simulink model "A1_acc"  (R2024a)
settings: Solver=ode45  StartTime=0.0  StopTime=80.0  MaxStep=0.001  RelTol=1e-3
values from neighbouring files (symbols this model uses):
  a = data(2)    [A1_10.m]    (also in problem6.m = 270)
  b = data(3)    [A1_10.m]    (also in problem6.m = 11000)
  kd = (0.155+3*p)/6.322    (= -0.0703416640304)    [problem8.m]    (also in problem815.m = -0.0703938627017)
  ki = p^3/6.322    (= -0.00126352515011)    [problem8.m]    (also in problem815.m = -0.00126561215755)
  kp = 3*p^2/(-6.322)    (= -0.0189623584309)    [problem8.m]    (also in problem815.m = -0.0189832332015)
  m = data(1)    [A1_10.m]    (also in problem6.m = 1740)
settings Model: Creator=jofr  LastModifiedBy=xiach
settings SolverCC: AlgebraicLoopSolver=TrustRegion
settings DataIOCC: LimitDataPoints=on  SaveFormat=Array  SignalLoggingSaveFormat=ModelDataLogs  ReturnWorkspaceOutputs=off
settings OptimizationCC: BlockReduction=off  BooleanDataType=off  LifeSpan=inf
settings DebuggingCC: SaveWithParameterizedLinksMsg=none  UnderspecifiedInitializationDetection=Classic  MergeDetectMultiDrivingBlocksExec=none  SignalResolutionControl=TryResolveAllWithWarning  MultiTaskDSMMsg=warning  MultiTaskCondExecSysMsg=none  UnconnectedInputMsg=warning  UnconnectedOutputMsg=warning  UnconnectedLineMsg=warning  SFUnexpectedBacktrackingDiag=warning  SFNoUnconditionalDefaultTransitionDiag=warning  SFExecutionAtInitializationDiag=none  ArithmeticOperatorsInVariantConditions=warning
settings HardwareCC: ProdBitPerPointer=32  ProdBitPerSizeT=32  ProdBitPerPtrDiffT=32  ProdLargestAtomicFloat=None  ProdIntDivRoundTo=Undefined  ProdEndianess=Unspecified  ProdWordSize=32  ProdHWDeviceType=32-bit Generic  TargetUnknown=on
settings ModelReferenceCC: EnableRefExpFcnMdlSchedulingChecks=on  PropagateSignalLabelsOutOfModel=off
settings SFSimCC: SimUseLocalCustomCode=off  CustomCodeUndefinedFunction=UseInterfaceOnly
settings RTWCC: RTWUseLocalCustomCode=off  GPUComputeCapability=3.5  DLArmComputeVersion=19.05
settings CodeAppCC: StateflowObjectComments=on
settings GRTTargetCC: TargetLangStandard=C89/C90 (ANSI)
settings ConfigComp: CovMetricSettings=dw  CovSaveCumulativeToWorkspaceVar=on  CovSaveSingleToWorkspaceVar=on  CovExternalEMLEnable=off

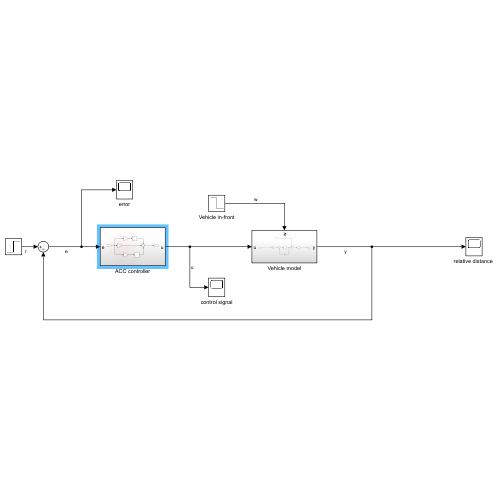
[thumbnail: Simulink's stored preview of the top-level diagram]
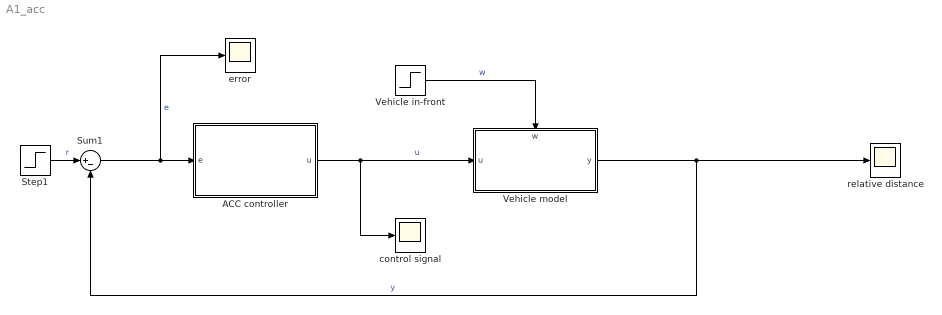
== system A1_acc ==
  ACC controller : Subsystem
  Step1 : Step  Time=10  Before=30  After=30  SampleTime=0
  Sum1 : Sum  Inputs=|+-
  Vehicle in-front : Step  Time=10  Before=25  After=15  SampleTime=0
  Vehicle model : Subsystem
      settings: PortSchema="{\"entries\":[{\"content\":{\"sides\":[{\"content\":{\"connectorIds\":[\"In1\"]},\"type\":\"ConnectorPlacement.EquallySpacedRectSide\",\"uuid\":\"8188ec2e-7b14-4fd6-ab55-7cea6e9f54e2\"},{\"content\":{\"connectorIds\":[\"Out1\"],\"side\":\"RIGHT\"},\"type\":\"ConnectorPlacement.EquallySpacedRectSide\",\"uuid\":\"403e2e46-1697-4bb6-98fa-f8a08edec7c4\"},{\"content\":{\"connectorIds\":[\"In2\"],\"side\":\"TOP\"},\"type\":\"ConnectorPlacement.EquallySpacedRectSide\",\"uuid\":\"1cc5364f-c05a-4d3f-ac94-5b665fe415b4\"},{\"content\":{\"connectorIds\":[],\"side\":\"HIDDEN\"},\"type\":\"ConnectorPlacement.EquallySpacedRectSide\",\"uuid\":\"4fc64fe0-eaad-4a3e-850d-8e1dbe967cca\"}]},\"type\":\"ConnectorPlacement.EquallySpacedConnector\",\"uuid\":\"84be3d81-93f1-400b-9ab2-2fcef574c47e\"}],\"packageUris\":[\"http://schema.mathworks.com/mf0/Connector/R2020b\"],\"version\":\"1.0\"}"
  control signal : Scope
  error : Scope
  "relative distance " : Scope
  wires:
  Sum1/1 -> ACC controller/1(e), error/1  "e"
  Step1/1 -> Sum1/1  "r"
  ACC controller/1(u) -> control signal/1, Vehicle model/1(u)  "u"
  Vehicle model/1(y) -> "relative distance "/1, Sum1/2  "y"
  Vehicle in-front/1 -> Vehicle model/2(w)  "w"

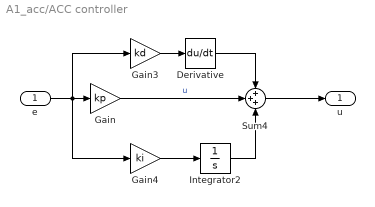
== system A1_acc/ACC controller ==
  e : Inport
  Derivative : Derivative
  Gain : Gain  Gain=kp
  Gain3 : Gain  Gain=kd
  Gain4 : Gain  Gain=ki
  Integrator2 : Integrator  InitialCondition=a*25/b
  Sum4 : Sum  Inputs=+++
  u : Outport
  wires:
  Integrator2/1 -> Sum4/3
  Sum4/1 -> u/1
  Derivative/1 -> Sum4/1
  e/1 -> Gain4/1, Gain3/1, Gain/1
  Gain/1 -> Sum4/2  "u"
  Gain4/1 -> Integrator2/1
  Gain3/1 -> Derivative/1

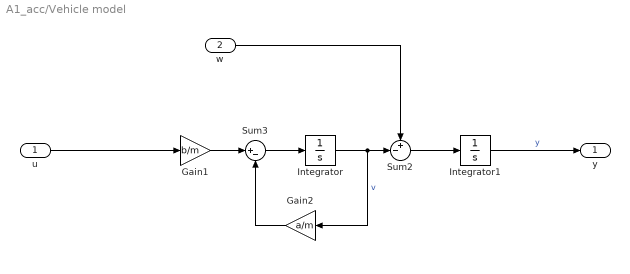
== system A1_acc/Vehicle model ==
  u : Inport
  w : Inport  Port=2
  Gain1 : Gain  Gain=b/m
  Gain2 : Gain  Gain=a/m
  Integrator : Integrator  InitialCondition=25
  Integrator1 : Integrator  InitialCondition=30
  Sum2 : Sum  Inputs=+-|
  Sum3 : Sum  Inputs=|+-
  y : Outport
  wires:
  w/1 -> Sum2/1
  u/1 -> Gain1/1
  Integrator1/1 -> y/1  "y"
  Integrator/1 -> Sum2/2, Gain2/1  "v"
  Gain2/1 -> Sum3/2
  Sum3/1 -> Integrator/1
  Sum2/1 -> Integrator1/1
  Gain1/1 -> Sum3/1
